simulink library "Fixed_Wing"  (R2023b)
settings: Solver=VariableStepAuto  StartTime=0.0  StopTime=10.0  RelTol=1e-3
values from neighbouring files (symbols this model uses):
  X8_lat_da_p_tf = X8_lat_p_tf(1)    [main.m]
  X8_lat_da_r_tf = X8_lat_r_tf(1)    [main.m]
  X8_lon_de_q_tf = X8_lon_q_tf(1)    [main.m]
  X8_lon_th_u_tf = X8_lon_u_tf(2)    [main.m]
  X8_lon_th_w_tf = X8_lon_w_tf(2)    [main.m]
undefined symbols (not defined in the file or in its folder): alpha, beta, env, init, k_phi, k_theta, k_Va, X8
libraries: $bdroot x16, simulink x2
(part 2 of 2)

== matlab function Fixed_Wing/Fixed Wing Formation Model with Wind Observer/Formation Error1/Geometry error  ==
  data: G_desired input; course_L input; G_error output; position_L input; position_F input
function G_error = geometry_error_generation(G_desired, course_L, position_L, position_F)
    G_error = [sin(course_L), -cos(course_L), 0 ; cos(course_L), sin(course_L), 0 ; 0, 0, -1]*(position_L - position_F) - G_desired;
end

== matlab function Fixed_Wing/Fixed Wing Formation Model with Wind Observer/Inertial to formation frame1 ==
  data: wind_i input; wind_f output; course_L input
function wind_f = fcn(wind_i, course_L)
    phi_L = 0; % assume zero first
    theta_L = 0; % assume zero first
    R_r = [1, 0     , 0     ;   
           0, cos(phi_L), -sin(phi_L);
           0, sin(phi_L),  cos(phi_L)];
    R_p = [cos(theta_L), 0, sin(theta_L);
             0     , 1, 0     ;
            -sin(theta_L), 0, cos(theta_L)];
    R_y = [cos(course_L), -sin(course_L), 0;
           sin(course_L),  cos(course_L), 0;
           0     ,  0     , 1];
    % inertial to body
    R = R_y*R_p*R_r;
    wind_b = transpose(R)* wind_i;
    % body to formation frame
    wind_f = [wind_b(2);-wind_b(1); wind_b(3)]; % wl, wf, wh
end

== matlab function Fixed_Wing/Inertial to formation frame ==
  data: wind_i input; wind_f output; course_L input
function wind_f = fcn(wind_i, course_L)
    phi_L = 0; % assume zero first
    theta_L = 0; % assume zero first
    R_r = [1, 0     , 0     ;   
           0, cos(phi_L), -sin(phi_L);
           0, sin(phi_L),  cos(phi_L)];
    R_p = [cos(theta_L), 0, sin(theta_L);
             0     , 1, 0     ;
            -sin(theta_L), 0, cos(theta_L)];
    R_y = [cos(course_L), -sin(course_L), 0;
           sin(course_L),  cos(course_L), 0;
           0     ,  0     , 1];
    % inertial to body
    R = R_y*R_p*R_r;
    wind_b = transpose(R)* wind_i;
    % body to formation frame
    wind_f = [wind_b(2);-wind_b(1); wind_b(3)]; % wl, wf, wh
end

== matlab function Fixed_Wing/Fixed Wing Formation Model with Wind Observer/Wind Observer/Position estimation ==
  data: L input; w_hat input; sigma input; velcocity_hat output; velocity_0 input
function velcocity_hat = velocityEstimation(L, w_hat, sigma, velocity_0)
    lambda1 = 1.5*L^(1/2);
    velcocity_hat = velocity_0 - lambda1*(abs(sigma).^(1/2).*sign(sigma))+ w_hat;
end

== matlab function Fixed_Wing/Fixed Wing Formation Model with Wind Observer/Wind Observer/Wind acceleration estimation ==
  data: L input; sigma input; w_a_hat output
function w_a_hat = WAEstimation(L, sigma)
    lamda0 = 1.1*L;
    w_a_hat = -lamda0*sign(sigma); 
end

== matlab function Fixed_Wing/kinematic(NED)_course/psi_generator  ==
  data: course input; psi output; Va input; theta input; wind input
function psi = fcn(course, Va, theta, wind)
    psi = course-asin(1/(Va*cos(theta))*wind(1:2)'*[-sin(course);cos(course)]);
end

== matlab function Fixed_Wing/NED -> ENU ==
  data: position_NED input; position_ENU output
function position_ENU = fcn(position_NED)
R_NED_ENU = [0 1 0;
             1 0 0;
             0 0 -1;];
position_ENU = R_NED_ENU* position_NED;
end

== matlab function Fixed_Wing/kinematic(NED)_course/Vg_generator ==
  data: psi input; Vg output; Va input; theta input; wind input
function Vg = fcn(psi, Va, theta, wind)
    Vw = norm(wind);
    Vg = sqrt(Va^2+Vw^2+2*Va*[cos(psi)*cos(theta);sin(psi)*cos(theta);-sin(theta)]'*wind);
end

== matlab function Fixed_Wing/Fixed Wing Model/Course error constraint [-pi, pi] ==
  data: err_course input; err_course output
function err_course = constraint(err_course)
    while err_course < -pi
        err_course = err_course + 2*pi;
        % err_lt_mpi = err_course
        % display("err < -pi", err_course);
    end
    while err_course > pi
        err_course = err_course - 2*pi;
        % err_gt_pi = err_course
        % display("err > pi", err_course);
    end
end

== matlab function Fixed_Wing/Fixed Wing Model/Course error constraint [-pi, pi]1 ==
  data: err_course input; err_course output
function err_course = constraint(err_course)
    while err_course < -pi
        err_course = err_course + 2*pi;
        % err_lt_mpi = err_course
        % display("err < -pi", err_course);
    end
    while err_course > pi
        err_course = err_course - 2*pi;
        % err_gt_pi = err_course
        % display("err > pi", err_course);
    end
end

== matlab function Fixed_Wing/kinematic(NED)_psi/Vg_generator ==
  data: psi input; Vg output; Va input; theta input; wind input
function Vg = fcn(psi, Va, theta, wind)
    Vw = norm(wind);
    Vg = sqrt(Va^2+Vw^2+2*Va*[cos(psi)*cos(theta);sin(psi)*cos(theta);-sin(theta)]'*wind);
end

== matlab function Fixed_Wing/kinematic(NED)_psi/course_generator  ==
  data: psi input; course output; Va input; Vg input; theta input; wind input; gamma output
function [course , gamma] = fcn(psi, Va, Vg, theta, wind)
    wn = wind(1);
    wd = wind(3);
    gamma = asin((Va*sin(theta)-wd)/Vg);
    course = acos((Va*cos(psi)*cos(theta)+wn)/(Vg*cos(gamma)));
end

== matlab function Fixed_Wing/Fixed Wing Model(Va,psi,theta)/Course error constraint [-pi, pi] ==
  data: err_course input; err_course output
function err_course = constraint(err_course)
    while err_course < -pi
        err_course = err_course + 2*pi;
        % err_lt_mpi = err_course
        % display("err < -pi", err_course);
    end
    while err_course > pi
        err_course = err_course - 2*pi;
        % err_gt_pi = err_course
        % display("err > pi", err_course);
    end
end

== matlab function Fixed_Wing/Fixed Wing Model(Va,psi,theta)/Course error constraint [-pi, pi]1 ==
  data: err_course input; err_course output
function err_course = constraint(err_course)
    while err_course < -pi
        err_course = err_course + 2*pi;
        % err_lt_mpi = err_course
        % display("err < -pi", err_course);
    end
    while err_course > pi
        err_course = err_course - 2*pi;
        % err_gt_pi = err_course
        % display("err > pi", err_course);
    end
end
